simulink model "withaqm_onehop"  (R2020b)
settings: Solver=VariableStepAuto  StartTime=0.0  StopTime=1000  RelTol=1e-3  EnableMultiTasking=on
InitFcn:
  | t = getCurrentTask();
  | if ~isempty(t)
  |     task_id = t.ID;
  | else
  |     task_id = 1;
  | end
values from neighbouring files (symbols this model uses):
  ml_model_config = [int32(10000), int32(3), int32(16),                        int32(1), int32(1), int32(4), int32(-5)]    [main.m]
  sim_vars = [ 0, 0.9                8, 1,               8, 1,               8, 1,               inf, inf, inf                rand(1,1)*100000             ]    [main.m]
undefined symbols (not defined in the file or in its folder): m, n
settings Model: SimulationMode=accelerator  Creator=The MathWorks, Inc.  LastModifiedBy=ssmos
settings DataIOCC: LimitDataPoints=on  SaveOperatingPoint=on  SaveFormat=StructureWithTime
settings OptimizationCC: LifeSpan=inf
settings DebuggingCC: AllowSymbolicDim=off  SFUnexpectedBacktrackingDiag=warning  SFNoUnconditionalDefaultTransitionDiag=warning  SFExecutionAtInitializationDiag=none  ArithmeticOperatorsInVariantConditions=warning
settings ModelReferenceCC: PropagateSignalLabelsOutOfModel=off
settings SFSimCC: SimUseLocalCustomCode=off  CustomCodeUndefinedFunction=UseInterfaceOnly
settings RTWCC: RTWUseLocalCustomCode=off
settings CodeAppCC: StateflowObjectComments=on
settings GRTTargetCC: TargetLangStandard=C89/C90 (ANSI)
settings ConfigComp: CovMetricSettings=dw  CovSaveCumulativeToWorkspaceVar=on  CovSaveSingleToWorkspaceVar=on  CovExternalEMLEnable=off  CovSFcnEnable=off

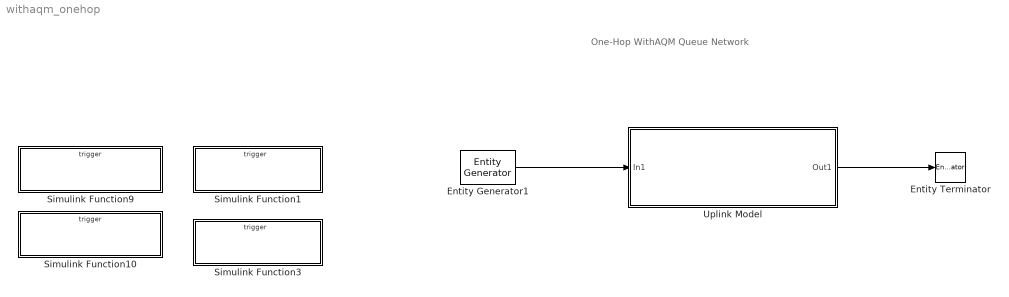
== system withaqm_onehop ==
  note: One-Hop WithAQM Queue Network
  Entity Generator1 : EntityGenerator  OutputPortMessageModes=m  TimeSource=MATLAB action  IntergenerationTimeAction=dt = getArrivalTime(sim_vars(1),sim_vars(2),sim_vars(12));  GenerateAction=|  AttributeName=starttime|queuen_uplink_bu|servern_uplink_bu|queuen_compute_bu|servern_compute_bu|queuen_downlink_bu|servern_downlink_bu|queuen_compute_bc|servern_compute_bc|queuen_downlink_bc|servern_downlink_bc|queuen_downlink_bd|servern_downlink_bd|queuetime_uplink|servicetime_uplink|queuetime_compute|servicetime_compute|queuetime_downlink|servicetime_downlink|endtime|drop_switch_port|service_dt  AttributeInitialValue=inf|-1|-1|-1|-1|-1|-1|-1|-1|-1|-1|-1|-1|inf|inf|inf|inf|inf|inf|inf|1|0  EntityType=Structured  EntityTypeName=Entity
      | entity.starttime = getCurrentTime();
      | 
      | entity.queuen_uplink_bu = getQueueNUplink();
      | entity.servern_uplink_bu = getServerNUplink();
  Entity Terminator : EntityTerminator  InputPortMessageModes=m  EntryAction=|
      | entity.endtime = getCurrentTime();
      | 
      | saveAttributes([entity.starttime;               ...
      |                 entity.queuen_uplink_bu;        ...
      |                 entity.servern_uplink_bu;       ...
      |                 entity.queuen_compute_bu;       ...
      |                 entity.servern_compute_bu;      ...
      |                 entity.queuen_downlink_bu;      ...
      |                 entity.servern_downlink_bu;     ...
      |                 entity.queuen_compute_bc;       ...
      |                 entity.servern_compute_bc;      ...
      |                 entity.queuen_downlink_bc;      ...
      |                 entity.servern_downlink_bc;     ...
      |                 entity.queuen_downlink_bd;      ...
      |                 entity.servern_downlink_bd;     ...
      |                 entity.queuetime_uplink;        ...
      |                 entity.servicetime_uplink;      ...
      |                 entity.queuetime_compute;       ...
      |                 entity.servicetime_compute;     ...
      |                 entity.queuetime_downlink;      ...
      |                 entity.servicetime_downlink;    ...
      |                 entity.endtime;                 ...
      |                 entitySys.id]);
  Simulink Function1 : Subsystem  TreatAsAtomicUnit=on
  Simulink Function10 : Subsystem  TreatAsAtomicUnit=on
  Simulink Function3 : Subsystem  TreatAsAtomicUnit=on
  Simulink Function9 : Subsystem  TreatAsAtomicUnit=on
  Uplink Model : Subsystem
  wires:
  Entity Generator1/1 -> Uplink Model/1(In1)
  Uplink Model/1(Out1) -> Entity Terminator/1

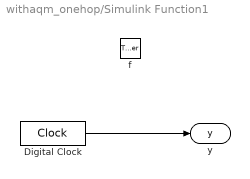
== system withaqm_onehop/Simulink Function1 ==
  f : TriggerPort  TriggerType=function-call  IsSimulinkFunction=on  FunctionName=getCurrentTime  VariantControl=(inherit)
  Digital Clock : DigitalClock  SampleTime=-1
  y : ArgOut  DisableCoverage=on  ArgumentName=y
  wires:
  Digital Clock/1 -> y/1

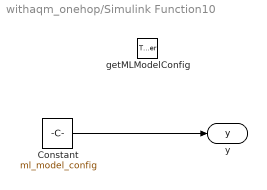
== system withaqm_onehop/Simulink Function10 ==
  getMLModelConfig : TriggerPort  TriggerType=function-call  IsSimulinkFunction=on  FunctionName=getMLModelConfig  VariantControl=(inherit)
  Constant : Constant  Value=ml_model_config
  y : ArgOut  DisableCoverage=on  OutDataTypeStr=int32  PortDimensions=7  ArgumentName=y
  wires:
  Constant/1 -> y/1

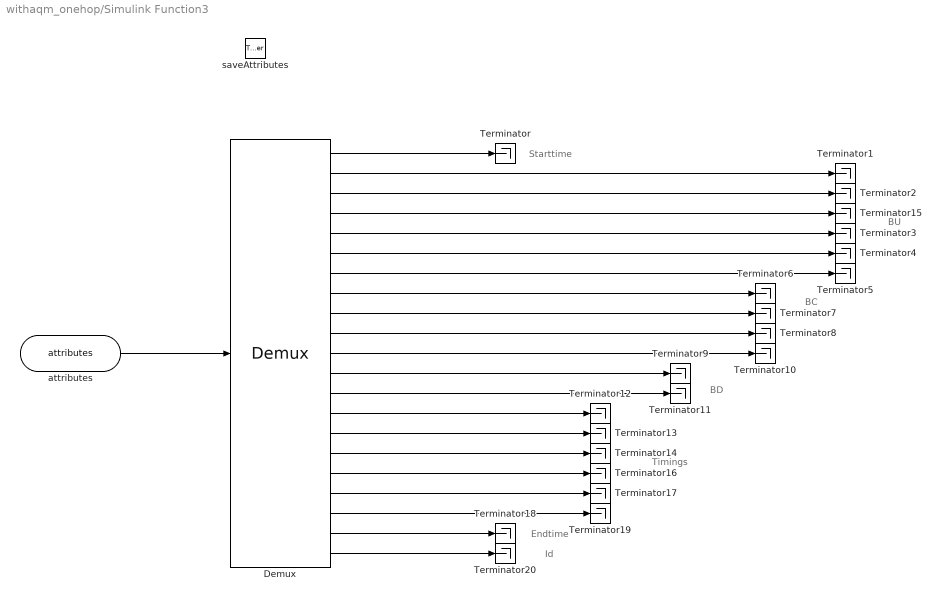
== system withaqm_onehop/Simulink Function3 ==
  note: Id
  note: Endtime
  note: Starttime
  note: Timings
  note: BU
  note: BC
  note: BD
  saveAttributes : TriggerPort  TriggerType=function-call  IsSimulinkFunction=on  FunctionName=saveAttributes  VariantControl=(inherit)
  Demux : Demux  Outputs=21
      settings: DisplayOption=none
  Terminator{,1..20} (21 alike) : Terminator
  attributes : ArgIn  DisableCoverage=on  PortDimensions=21  ArgumentName=attributes
  wires:
  attributes/1 -> Demux/1
  Demux/1 -> Terminator/1
  Demux/2 -> Terminator1/1
  Demux/3 -> Terminator2/1
  Demux/7 -> Terminator5/1
  Demux/5 -> Terminator3/1
  Demux/6 -> Terminator4/1
  Demux/8 -> Terminator6/1
  Demux/4 -> Terminator15/1
  Demux/9 -> Terminator7/1
  Demux/10 -> Terminator8/1
  Demux/11 -> Terminator10/1
  Demux/12 -> Terminator9/1
  Demux/13 -> Terminator11/1
  Demux/14 -> Terminator12/1
  Demux/15 -> Terminator13/1
  Demux/16 -> Terminator14/1
  Demux/17 -> Terminator16/1
  Demux/18 -> Terminator17/1
  Demux/19 -> Terminator19/1
  Demux/20 -> Terminator18/1
  Demux/21 -> Terminator20/1

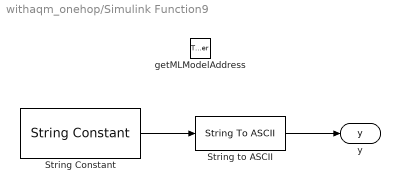
== system withaqm_onehop/Simulink Function9 ==
  getMLModelAddress : TriggerPort  TriggerType=function-call  IsSimulinkFunction=on  FunctionName=getMLModelAddress  VariantControl=(inherit)
  String Constant : StringConstant  String=ml_model_address
  String to ASCII : StringToASCII  OutputVectorSize=500
  y : ArgOut  DisableCoverage=on  OutDataTypeStr=uint8  PortDimensions=500  ArgumentName=y
  wires:
  String Constant/1 -> String to ASCII/1
  String to ASCII/1 -> y/1

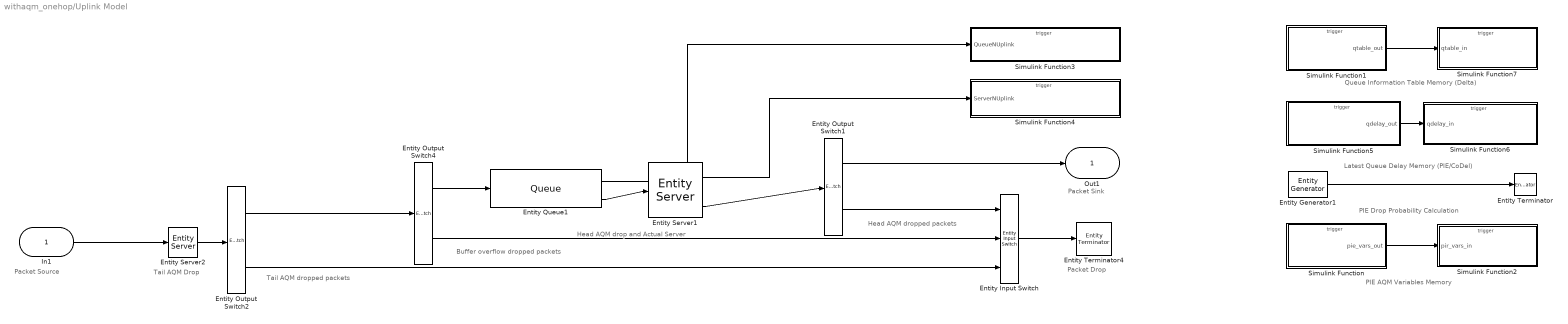
== system withaqm_onehop/Uplink Model ==
  note: Head AQM drop and Actual Server
  note: Head AQM dropped packets
  note: Buffer overflow dropped packets
  note: Tail AQM Drop
  note: Tail AQM dropped packets
  note: Packet Drop
  note: Packet Sink
  note: Packet Source
  note: Queue Information Table Memory (Delta)
  note: PIE Drop Probability Calculation
  note: PIE AQM Variables Memory
  note: Latest Queue Delay Memory (PIE/CoDel)
  In1 : Inport
  Entity Input Switch : EntityInputSwitch  InputPortMessageModes=m,m,m  OutputPortMessageModes=m  NumberInputPorts=3
      settings: InputPortMap=u1,u2,u3
  Entity Output Switch1 : EntityOutputSwitch  InputPortMessageModes=m  OutputPortMessageModes=m,m  SwitchingCriterion=From attribute  SwitchAttributeName=drop_switch_port
  Entity Output Switch2 : EntityOutputSwitch  InputPortMessageModes=m  OutputPortMessageModes=m,m  SwitchingCriterion=From attribute  SwitchAttributeName=drop_switch_port
  Entity Output Switch4 : EntityOutputSwitch  InputPortMessageModes=m  OutputPortMessageModes=m,m  SwitchAttributeName=drop_at_source
  Entity Generator1 : EntityGenerator  OutputPortMessageModes=m  TimeSource=MATLAB action  IntergenerationTimeAction=|  GenerateEntityAtSimulationStart=off  EntityType=Structured  EntityTypeName=PIE_bell
      | if (aqm_params(1) == 1)
      |     T_UPDATE = aqm_params(6);
      |     dt = T_UPDATE;
      | else
      |     dt = inf;
  Entity Queue1 : Queue  InputPortMessageModes=m  OutputPortMessageModes=n,m  Capacity=sim_vars(9)  NumberEntitiesInBlock=on
      settings: OutputPortMap=o1,o5
  Entity Server1 : EntityServer  InputPortMessageModes=m  OutputPortMessageModes=n,m  Capacity=1  ServiceTimeSource=MATLAB action  ServiceTimeAction=|  EntryAction=|  ServiceCompleteAction=|  NumberEntitiesInBlock=on
      ServiceTimeAction=|
      | % if supposed to be dropped
      | if (entity.drop_switch_port == 2) 
      |     dt = 0;
      | else
      |     % entity.service_dt is set in event actions entry
      |     dt = entity.service_dt;
      | end
      EntryAction=|
      | %%%%%%%%%%%%%%%%%%%%%%%%%%%%%%%%%%%%%%%%%%%%%%%%%%%%%%%%%%%%%%
      | %% Non-AQM Stuff %%%%%%%%%%%%%%%%%%%%%%%%%%%%%%%%%%%%%%%%%%%%%
      | 
      | % update packet's queue timestamp
      | entity.queuetime_uplink = getCurrentTime();
      | % define the packet drop variable
      | drop_the_packet = 0;
      | 
      | %%%%%%%%%%%%%%%%%%%%%%%%%%%%%%%%%%%%%%%%%%%%%%%%%%%%%%%%%%%%%%
      | %% Delta-AQM: (1) Update Queue Table Latency Budgets %%%%%%%%%
      | qt = []
      | if aqm_params(1) == 3
      | 
      |     qt = getQueueInfoTable();
      |     now = getCurrentTime();
      |     nrow = sum(qt(:,3)==1);
      | 
      |     % update the table
      |     for r=1:nrow
      |         % Table format: [update_time, latency_budget]
      |         time_dif = now - qt(r,1);
      |         qt(r,2) = qt(r,2)-time_dif;
      |         qt(r,1) = now;
      |     end
      | 
      | end
      | 
      | %%%%%%%%%%%%%%%%%%%%%%%%%%%%%%%%%%%%%%%%%%%%%%%%%%%%%%%%%%%%%%
      | %% Delta-AQM: (2) Drop the Packet %%%%%%%%%%%%%%%%%%%%%%%%%%%%
      | if aqm_params(1) == 3
      |     
      |     % task_id is set at the model properties, init callback function
      |     drop_the_packet = dequeueDelta( qt, ...
      |                                     getMLModelConfig(), ...
      |                                     getMLModelAddress(), ...
      |                                     task_id);
      |     
      |     %disp('-')
      |     %disp(entity.drop_at_source)
      |     %disp(qt(1:nrow,:))
      |     %disp('-')
      | end
      | 
      | %%%%%%%%%%%%%%%%%%%%%%%%%%%%%%%%%%%%%%%%%%%%%%%%%%%%%%%%%%%%%%
      | %% PIE and CoDel: calculate queue delay and save %%%%%%%%%%%%%
      | if aqm_params(1) == 2 || aqm_params(1) == 1
      |     
      |     latest_queue_delay = entity.queuetime_uplink - entity.starttime;
      |     setLatestQueueDelay(latest_queue_delay);
      |     
      | end
      | 
      | %%%%%%%%%%%%%%%%%%%%%%%%%%%%%%%%%%%%%%%%%%%%%%%%%%%%%%%%%%%%%%
      | %% Codel AQM %%%%%%%%%%%%%%%%%%%%%%%%%%%%%%%%%%%%%%%%%%%%%%%%%
      | if aqm_params(1) == 2
      |     
      |     INTERVAL = aqm_params(6);
      |     DELAY_TARGET = aqm_params(7);
      |     drop_the_packet = dequeueCoDel(latest_queue_delay,getCurrentTime(),INTERVAL,DELAY_TARGET);
      |     
      | end
      | 
      | %%%%%%%%%%%%%%%%%%%%%%%%%%%%%%%%%%%%%%%%%%%%%%%%%%%%%%%%%%%%%%
      | %% PIE AQM %%%%%%%%%%%%%%%%%%%%%%%%%%%%%%%%%%%%%%%%%%%%%%%%%%%
      | if aqm_params(1) == 1
      |     
      |     QDELAY_REF = aqm_params(4);
      |     MEAN_PKTSIZE = aqm_params(5);
      |     T_UPDATE = aqm_params(6);
      |     ALPHA = aqm_params(7);
      |     BETA = aqm_params(8);
      | 
      |     [drop_prob,qdelay_old] = updateDropProbPIE(latest_queue_delay,ALPHA,BETA,QDELAY_REF,T_UPDATE, getCurrentTime());
      |     setPIEVariables([drop_prob;qdelay_old]);
      | 
      | end
      | 
      | %%%%%%%%%%%%%%%%%%%%%%%%%%%%%%%%%%%%%%%%%%%%%%%%%%%%%%%%%%%%%%
      | %% Delta-AQM: (3) Remove the First Packet from Queue Table %%%
      | if aqm_params(1) == 3
      |     
      |     QUEUE_INFO_TABLE_SIZE = aqm_params(11);
      |     
      |     % Then, remove the first row and add zero entry at the tail
      |     [s,m] = size(qt);
      |     new_qt = [];
      |     for r = 2:s % skip the first
      |         new_qt = [new_qt;qt(r,:)];
      |     end
      |     new_qt = [new_qt;[0,0,0]];
      |     
      |     % save the new table
      |     setQueueInfoTable(new_qt(1:QUEUE_INFO_TABLE_SIZE,:));
      | 
      | end
      | 
      | 
      | %%%%%%%%%%%%%%%%%%%%%%%%%%%%%%%%%%%%%%%%%%%%%%%%%%%%%%%%%%%%%%
      | %% Calculate service DT %%%%%%%%%%%%%%%%%%%%%%%%%%%%%%%%%%%%%%
      | 
      | dt = getServiceTimeUplink(sim_vars(3),sim_vars(4),sim_vars(12));
      | if drop_the_packet == 1
      |     entity.service_dt = 0;
      |     entity.drop_switch_port = 2;
      | else
      |     entity.service_dt = dt;
      |     entity.drop_switch_port = 1;
      | end
      ServiceCompleteAction=|
      | %% update service time
      | % if supposed to be dropped
      | if (entity.drop_switch_port == 2)
      |     entity.servicetime_uplink = inf;
      | else
      |     entity.servicetime_uplink = getCurrentTime();
      | end
      settings: OutputPortMap=o1,o9
  Entity Server2 : EntityServer  InputPortMessageModes=m  OutputPortMessageModes=m  Capacity=1  ServiceTimeSource=MATLAB action  ServiceTimeAction=dt = 0;  EntryAction=|
      | %%%%%%%%%%%%%%%%%%%%%%%%%%%%%%%%%%%%%%%%%%%%%%%%
      | %% PIE AQM Dropping Process %%%%%%%%%%%%%%%%%%%%
      | 
      | if aqm_params(1)==1 % if PIE is enabled
      |     
      |     % pie implementation
      |     QDELAY_REF = aqm_params(4);
      |     MEAN_PKTSIZE = aqm_params(5);
      | 
      |     pie_vars = getPIEVariables();
      |     drop_prob = pie_vars(1);
      |     qdelay_old = pie_vars(2);
      | 
      |     queue_length = getQueueNUplink();
      |     server_length = getServerNUplink();
      | 
      |     drop_the_packet = enqueuePIE(drop_prob,qdelay_old,queue_length, ...
      |                                  MEAN_PKTSIZE,QDELAY_REF,sim_vars(12));
      |     if drop_the_packet == 1
      |         entity.drop_switch_port = 2;
      |     else
      |         entity.drop_switch_port = 1;
      |     end
      |     
      | end
  Entity Terminator : EntityTerminator  InputPortMessageModes=m  EntryAction=|
      | if (aqm_params(1) == 1)
      |     
      |     QDELAY_REF = aqm_params(4);
      |     MEAN_PKTSIZE = aqm_params(5);
      |     T_UPDATE = aqm_params(6);
      |     ALPHA = aqm_params(7);
      |     BETA = aqm_params(8);
      |     
      |     latest_queue_delay = getLatestQueueDelay();
      |     
      |     [drop_prob,qdelay_old] = updateDropProbPIEInterval(latest_queue_delay,ALPHA,BETA,QDELAY_REF);
      |     setPIEVariables([drop_prob;qdelay_old]);
      |     
      | end
  Entity Terminator4 : EntityTerminator  InputPortMessageModes=m  EntryAction=|
      | saveAttributes([entity.starttime;               ...
      |                 entity.queuen_uplink_bu;        ...
      |                 entity.servern_uplink_bu;       ...
      |                 entity.queuen_compute_bu;       ...
      |                 entity.servern_compute_bu;      ...
      |                 entity.queuen_downlink_bu;      ...
      |                 entity.servern_downlink_bu;     ...
      |                 entity.queuen_compute_bc;       ...
      |                 entity.servern_compute_bc;      ...
      |                 entity.queuen_downlink_bc;      ...
      |                 entity.servern_downlink_bc;     ...
      |                 entity.queuen_downlink_bd;      ...
      |                 entity.servern_downlink_bd;     ...
      |                 entity.queuetime_uplink;        ...
      |                 entity.servicetime_uplink;      ...
      |                 entity.queuetime_compute;       ...
      |                 entity.servicetime_compute;     ...
      |                 entity.queuetime_downlink;      ...
      |                 entity.servicetime_downlink;    ...
      |                 entity.endtime;                 ...
      |                 entitySys.id]);
  Simulink Function : Subsystem  TreatAsAtomicUnit=on
  Simulink Function1 : Subsystem  TreatAsAtomicUnit=on
  Simulink Function2 : Subsystem  TreatAsAtomicUnit=on
  Simulink Function3 : Subsystem  TreatAsAtomicUnit=on
  Simulink Function4 : Subsystem  TreatAsAtomicUnit=on
  Simulink Function5 : Subsystem  TreatAsAtomicUnit=on
  Simulink Function6 : Subsystem  TreatAsAtomicUnit=on
  Simulink Function7 : Subsystem  TreatAsAtomicUnit=on
  Out1 : Outport
  wires:
  Entity Queue1/1 -> Simulink Function3/1(QueueNUplink)
  Entity Server1/1 -> Simulink Function4/1(ServerNUplink)
  Entity Output Switch4/1 -> Entity Queue1/1
  Entity Queue1/2 -> Entity Server1/1
  Entity Output Switch1/2 -> Entity Input Switch/1
  Entity Server1/2 -> Entity Output Switch1/1
  Entity Output Switch1/1 -> Out1/1
  Entity Output Switch4/2 -> Entity Input Switch/2
  Entity Input Switch/1 -> Entity Terminator4/1
  In1/1 -> Entity Server2/1
  Entity Server2/1 -> Entity Output Switch2/1
  Entity Output Switch2/1 -> Entity Output Switch4/1
  Entity Output Switch2/2 -> Entity Input Switch/3
  Simulink Function/1(pie_vars_out) -> Simulink Function2/1(pir_vars_in)
  Simulink Function1/1(qtable_out) -> Simulink Function7/1(qtable_in)
  Entity Generator1/1 -> Entity Terminator/1
  Simulink Function5/1(qdelay_out) -> Simulink Function6/1(qdelay_in)

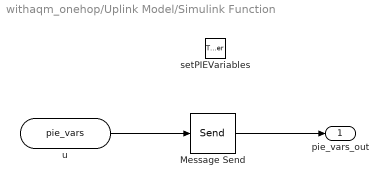
== system withaqm_onehop/Uplink Model/Simulink Function ==
  setPIEVariables : TriggerPort  TriggerType=function-call  IsSimulinkFunction=on  FunctionName=setPIEVariables  FunctionVisibility=scoped  VariantControl=(inherit)
  Message Send : Send  OutputPortMessageModes=m
  u : ArgIn  DisableCoverage=on  PortDimensions=2  ArgumentName=pie_vars
  pie_vars_out : Outport  InitialOutput=[0,0]  VectorParamsAs1DForOutWhenUnconnected=off
  wires:
  u/1 -> Message Send/1
  Message Send/1 -> pie_vars_out/1

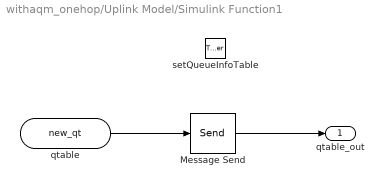
== system withaqm_onehop/Uplink Model/Simulink Function1 ==
  setQueueInfoTable : TriggerPort  TriggerType=function-call  IsSimulinkFunction=on  FunctionName=setQueueInfoTable  FunctionVisibility=scoped  VariantControl=(inherit)
  Message Send : Send  OutputPortMessageModes=m
  qtable : ArgIn  DisableCoverage=on  PortDimensions=[100,3]  ArgumentName=new_qt
  qtable_out : Outport  InitialOutput=zeros(100,3)  VectorParamsAs1DForOutWhenUnconnected=off
  wires:
  qtable/1 -> Message Send/1
  Message Send/1 -> qtable_out/1

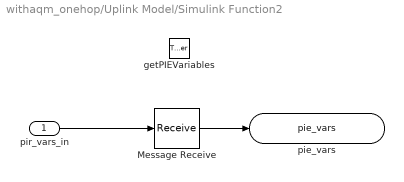
== system withaqm_onehop/Uplink Model/Simulink Function2 ==
  pir_vars_in : Inport
  getPIEVariables : TriggerPort  TriggerType=function-call  IsSimulinkFunction=on  FunctionName=getPIEVariables  FunctionVisibility=scoped  VariantControl=(inherit)
  Message Receive : Receive  InputPortMessageModes=m  QueueOverwriting=on  QueueLength=1  InitialValue=[0,0]
  pie_vars : ArgOut  DisableCoverage=on  PortDimensions=2  ArgumentName=pie_vars
  wires:
  pir_vars_in/1 -> Message Receive/1
  Message Receive/1 -> pie_vars/1

== system withaqm_onehop/Uplink Model/Simulink Function3 ==
  QueueNUplink : Inport
  getQueueNUplink : TriggerPort  TriggerType=function-call  IsSimulinkFunction=on  FunctionName=getQueueNUplink  VariantControl=(inherit)
  QueueNCompute : ArgOut  DisableCoverage=on  ArgumentName=QueueNUplink
  wires:
  QueueNUplink/1 -> QueueNCompute/1

== system withaqm_onehop/Uplink Model/Simulink Function4 ==
  ServerNUplink : Inport
  getServerNUplink : TriggerPort  TriggerType=function-call  IsSimulinkFunction=on  FunctionName=getServerNUplink  VariantControl=(inherit)
  QueueNCompute : ArgOut  DisableCoverage=on  ArgumentName=ServerNUplink
  wires:
  ServerNUplink/1 -> QueueNCompute/1

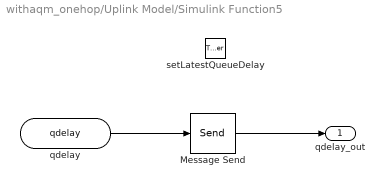
== system withaqm_onehop/Uplink Model/Simulink Function5 ==
  setLatestQueueDelay : TriggerPort  TriggerType=function-call  IsSimulinkFunction=on  FunctionName=setLatestQueueDelay  FunctionVisibility=scoped  VariantControl=(inherit)
  Message Send : Send  OutputPortMessageModes=m
  qdelay : ArgIn  DisableCoverage=on  ArgumentName=qdelay
  qdelay_out : Outport  InitialOutput=[0]  VectorParamsAs1DForOutWhenUnconnected=off
  wires:
  qdelay/1 -> Message Send/1
  Message Send/1 -> qdelay_out/1

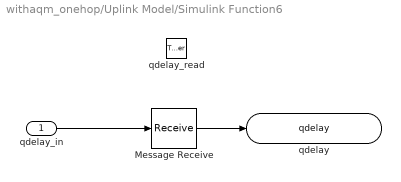
== system withaqm_onehop/Uplink Model/Simulink Function6 ==
  qdelay_in : Inport
  qdelay_read : TriggerPort  TriggerType=function-call  IsSimulinkFunction=on  FunctionName=getLatestQueueDelay  FunctionVisibility=scoped  VariantControl=(inherit)
  Message Receive : Receive  InputPortMessageModes=m  QueueOverwriting=on  QueueLength=1  InitialValue=[0]
  qdelay : ArgOut  DisableCoverage=on  ArgumentName=qdelay
  wires:
  qdelay_in/1 -> Message Receive/1
  Message Receive/1 -> qdelay/1

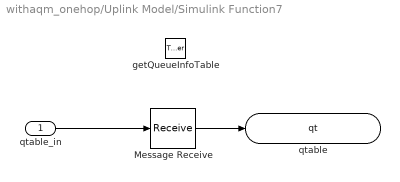
== system withaqm_onehop/Uplink Model/Simulink Function7 ==
  qtable_in : Inport
  getQueueInfoTable : TriggerPort  TriggerType=function-call  IsSimulinkFunction=on  FunctionName=getQueueInfoTable  FunctionVisibility=scoped  VariantControl=(inherit)
  Message Receive : Receive  InputPortMessageModes=m  QueueOverwriting=on  QueueLength=1  InitialValue=zeros(100,3)
  qtable : ArgOut  DisableCoverage=on  PortDimensions=[100,3]  ArgumentName=qt
  wires:
  qtable_in/1 -> Message Receive/1
  Message Receive/1 -> qtable/1
